simulink model "L3_Q1_Sim"  (R2015a)
settings: Solver=ode3  StartTime=0.0  StopTime=tf  FixedStep=t_step  RelTol=1e-3
values from neighbouring files (symbols this model uses):
  a = 0.01    [L3_Q1.m]    (also in L3_Q2.m)
  am = 0.1    [L3_Q1.m]
  av0_hat = bm / b0_hat    (= 0.1)    [L3_Q1.m]
  ax0_hat = (a0_hat - am) / b0_hat    (= -0.08)    [L3_Q1.m]
  b = 2    [L3_Q1.m]    (also in L3_Q2.m)
  bm = 0.1    [L3_Q1.m]
  gamma = 0.1    [L3_Q1.m]
  K0 = -log(0.01)/0.5    [L3_Q1.m]    (also in L3_Q2.m)
  T_ref = 2    [L3_Q1.m]    (also in L3_Q2.m)
settings Model: Creator=Marcelo  LastModifiedBy=Marcelo

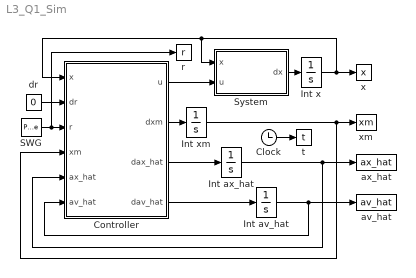
== system L3_Q1_Sim ==
  Clock : Clock
  Controller : MATLAB Function  TreatAsAtomicUnit=on
  Int av_hat : Integrator  InitialCondition=av0_hat
  Int ax_hat : Integrator  InitialCondition=ax0_hat
  Int x : Integrator
  Int xm : Integrator
  SWG : DiscretePulseGenerator  PulseType=Time based  Period=T_ref  PulseWidth=50
  System : MATLAB Function  TreatAsAtomicUnit=on
  av_hat : ToWorkspace  VariableName=av_hat  SampleTime=-1
  ax_hat : ToWorkspace  VariableName=ax_hat  SampleTime=-1
  dr : Constant  Value=0
  r : ToWorkspace  VariableName=r  SampleTime=-1
  t : ToWorkspace  VariableName=t  SampleTime=-1
  x : ToWorkspace  VariableName=x  SampleTime=-1
  xm : ToWorkspace  VariableName=xm  SampleTime=-1
  wires:
  System/1(dx) -> Int x/1
  Int x/1 -> x/1, System/1(x), Controller/1(x)
  Controller/1(u) -> System/2(u)
  Controller/2(dxm) -> Int xm/1
  Controller/3(dax_hat) -> Int ax_hat/1
  Controller/4(dav_hat) -> Int av_hat/1
  Int av_hat/1 -> av_hat/1, Controller/6(av_hat)
  Int ax_hat/1 -> ax_hat/1, Controller/5(ax_hat)
  Int xm/1 -> xm/1, Controller/4(xm)
  Clock/1 -> t/1
  SWG/1 -> r/1, Controller/3(r)
  dr/1 -> Controller/2(dr)

== matlab function L3_Q1_Sim/Controller ==
  data: u output; dxm output; x input; dr input; r input; xm input; ax_hat input; av_hat input; dax_hat output; dav_hat output; am parameter; bm parameter; gamma parameter; K0 parameter
function [u, dxm, dax_hat, dav_hat] = fcn(x, dr, r, xm, ax_hat, av_hat, am, bm, gamma, K0)
vm = dr - K0 * (xm - r);
um = (am*r + vm) / bm;
dxm = -am*xm + bm*um;

z = x - xm;
dax_hat = - gamma * z * x;
dav_hat = - gamma * z * um;
u = ax_hat*x + av_hat*um;

== matlab function L3_Q1_Sim/System ==
  data: x input; u input; dx output; a parameter; b parameter
function dx = fcn(x, u, a, b)
dx = -a*x + b*u;
